simulink model "CommandeClassique"  (R2018a)
settings: Solver=ode4  StartTime=0.0  StopTime=4  FixedStep=1e-5  RelTol=1e-3  EnableMultiTasking=on
values from neighbouring files (symbols this model uses):
  c1 = 0.5176    [Parameters.m]
  c2 = 116    [Parameters.m]
  c3 = 0.4    [Parameters.m]
  c4 = 5    [Parameters.m]
  c5 = 21    [Parameters.m]
  c6 = 0.0068    [Parameters.m]
  Cf = 2e-3    (= 0.002)    [Parameters.m]
  F = (Ft/(G^2))+Fg    (= 0.00731299039781)    [Parameters.m]
  Fsn = 50    [Parameters.m]
  G = 5.4    [Parameters.m]
  J = (Jt/(G^2))+Jg    (= 0.313940329218)    [Parameters.m]
  ki_c = 10*Rr/tou1    (= 620000)    [Parameters.m]
  ki_mppt = J*(wn^2)    (= 10.6826917581)    [Parameters.m]
  ki_p = 1/tou2    (= 100)    [Parameters.m]
  kif = 3*Rf/trf    (= 300)    [Parameters.m]
  kiv_voc = Cf*wn1^2    (= 480.2)    [Parameters.m]
  kp_c = (Lr-((Msr^2)/Ls))/tou1    (= 857.142857143)    [Parameters.m]
  kp_mppt = 2*xi*wn*J    (= 12.8192301097)    [Parameters.m]
  kp_p = tou1/tou2    (= 0.001)    [Parameters.m]
  kpf = 3*Lf/trf    (= 14)    [Parameters.m]
  kpv_voc = 2*ksi1*Cf*wn1    (= 2.548)    [Parameters.m]
  Lf = 0.014    [Parameters.m]
  Lr = 0.081    [Parameters.m]
  Ls = 0.084    [Parameters.m]
  Msr = 0.078    [Parameters.m]
  p = 2    [Parameters.m]
  R = 3    [Parameters.m]
  Rf = 0.3    [Parameters.m]
  rou = 1.225    [Parameters.m]
  s = pi*(R^2)    (= 28.2743338823)    [Parameters.m]
  sigm = (1-((Msr^2)/(Lr*Ls)))    (= 0.10582010582)    [Parameters.m]
  Tr = Lr/Rr    (= 0.13064516129)    [Parameters.m]
  Ts = Ls/Rs    (= 0.184615384615)    [Parameters.m]
  Vs = 380    [Parameters.m]
  Vsn = E/sqrt(3)    [Parameters.m]
  ws = Fsn*pi*2    (= 314.159265359)    [Parameters.m]
undefined symbols (not defined in the file or in its folder): fc
libraries: simulink x26, powerlib_extras x1
settings Model: Creator=HP  LastModifiedBy=Admin
settings DataIOCC: LimitDataPoints=on  SaveFormat=Array  SignalLoggingSaveFormat=ModelDataLogs
settings OptimizationCC: ExpressionDepthLimit=2147483647  LifeSpan=inf
settings DebuggingCC: UnderspecifiedInitializationDetection=Classic  MergeDetectMultiDrivingBlocksExec=none  SolverPrmCheckMsg=warning  FcnCallInpInsideContextMsg=warning  StateNameClashWarn=warning  SFUnexpectedBacktrackingDiag=warning  SFNoUnconditionalDefaultTransitionDiag=warning  SFExecutionAtInitializationDiag=none
settings HardwareCC: ProdBitPerPointer=32  ProdBitPerSizeT=32  ProdBitPerPtrDiffT=32  ProdLargestAtomicFloat=None  ProdIntDivRoundTo=Undefined  ProdEndianess=Unspecified  ProdWordSize=32  ProdHWDeviceType=32-bit Generic
settings ModelReferenceCC: PropagateSignalLabelsOutOfModel=off
settings CodeAppCC: StateflowObjectComments=on
settings GRTTargetCC: TargetLangStandard=C89/C90 (ANSI)  GeneratePreprocessorConditionals=Disable all  CombineOutputUpdateFcns=off  GRTInterface=on
settings ConfigComp: CovMetricSettings=dw  CovHtmlReporting=on  CovSaveCumulativeToWorkspaceVar=on  CovSaveSingleToWorkspaceVar=on  CovExternalEMLEnable=off

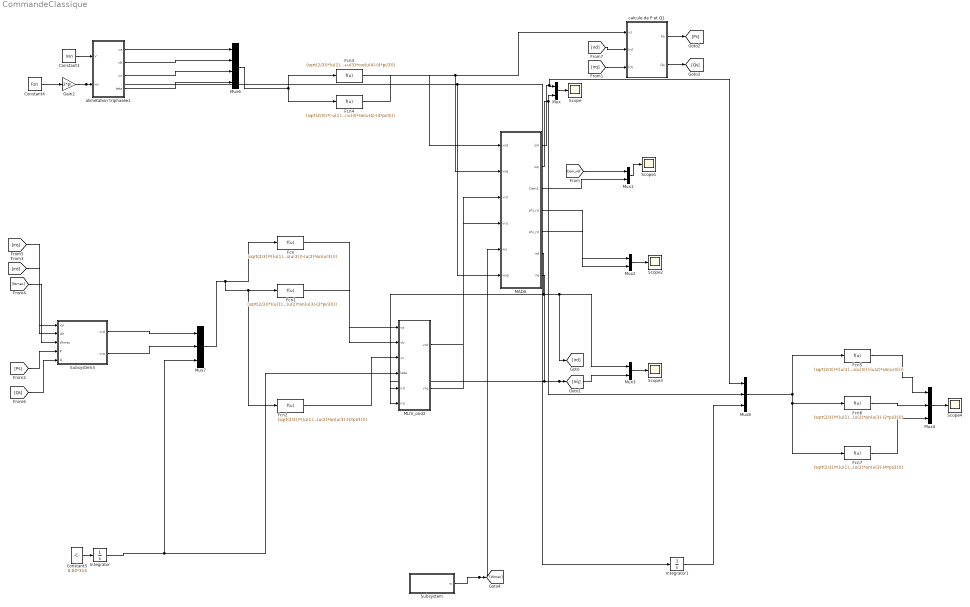
== system CommandeClassique ==
  Constant3 : Constant  Value=Vsn
  Constant4 : Constant  Value=Fsn
  Constant5 : Constant  Value=0.04*314
  Fcn : Fcn  Expr=(sqrt(2/3))*((u(1)*cos(u(3)))-(u(2)*sin(u(3))))
  Fcn1 : Fcn  Expr=(sqrt(2/3))*((u(1)*cos(u(3)-(2*pi/3)))-(u(2)*sin(u(3)-(2*pi/3))))
  Fcn2 : Fcn  Expr=(sqrt(2/3))*((u(1)*cos(u(3)-(4*pi/3)))-(u(2)*sin(u(3)-(4*pi/3))))
  Fcn3 : Fcn  Expr=(sqrt(2/3))*(u(1)*cos(u(4))+u(2)*cos(u(4)-(2*pi/3))+u(3)*cos(u(4)-(4*pi/3)))
  Fcn4 : Fcn  Expr=(sqrt(2/3))*(-u(1)*sin(u(4))-u(2)*sin(u(4)-(2*pi/3))-u(3)*sin(u(4)-(4*pi/3)))
  Fcn5 : Fcn  Expr=(sqrt(2/3))*((u(1)*cos(u(3)))-(u(2)*sin(u(3))))
  Fcn6 : Fcn  Expr=(sqrt(2/3))*((u(1)*cos(u(3)-(2*pi/3)))-(u(2)*sin(u(3)-(2*pi/3))))
  Fcn7 : Fcn  Expr=(sqrt(2/3))*((u(1)*cos(u(3)-(4*pi/3)))-(u(2)*sin(u(3)-(4*pi/3))))
  Gain2 : Gain  Gain=2*pi
  Integrator : Integrator
  Integrator1 : Integrator
  MADA : Subsystem
  MLIV_ond2 : Subsystem
  Mux{,1..3} (4 alike) : Mux  Inputs=2
  Mux4 : Mux  Inputs=3
  Mux6 : Mux
  Mux7 : Mux  Inputs=3
  Mux8 : Mux  Inputs=3
  Scope{,1..4} (5 alike) : Scope
  Subsystem : Subsystem
  Subsystem3 : Subsystem
  alimetation triphasée1 : Subsystem
  calcule de P et Q1 : Subsystem
  wires:
  Constant4/1 -> Gain2/1
  Gain2/1 -> MADA/6(wsp), Integrator1/1, alimetation triphasée1/2(ws)
  Constant3/1 -> alimetation triphasée1/1(V)
  Fcn3/1 -> MADA/1(vsd)
  Fcn4/1 -> calcule de P et Q1/1(vs), MADA/2(vsq)
  [irq] -> Subsystem3/1(iqr)
  [ird] -> Subsystem3/2(idr)
  [Wmec] -> Subsystem3/3(Wmec)
  [Ps] -> Subsystem3/4(P)
  Constant5/1 -> Integrator/1
  MADA/6(ird) -> Mux3/1, [ird], MLIV_ond2/5(ird)
  MADA/7(irq) -> Mux3/2, [irq], MLIV_ond2/6(irq)
  calcule de P et Q1/1(Ps) -> [Ps]
  calcule de P et Q1/2(Qs) -> [Qs]
  Fcn/1 -> MLIV_ond2/1(va)
  Fcn1/1 -> MLIV_ond2/2(vb)
  Fcn2/1 -> MLIV_ond2/3(vc)
  MLIV_ond2/1(vrd) -> MADA/3(vrd)
  MLIV_ond2/2(vrq) -> MADA/4(vrq)
  [ird] -> calcule de P et Q1/2(Ird)
  [irq] -> calcule de P et Q1/3(Irq)
  [Qs] -> Subsystem3/5(Q)
  MADA/3(Cem1) -> Mux1/2
  Subsystem/1(w) -> [Wmec], MADA/5(w1)
  Mux/1 -> Scope/1
  Mux1/1 -> Scope1/1
  [Cem_ref] -> Mux1/1
  Mux2/1 -> Scope2/1
  MADA/5(phi_rd) -> Mux2/1
  MADA/4(phi_rq) -> Mux2/2
  Mux3/1 -> Scope3/1
  Fcn6/1 -> Mux4/2
  Fcn7/1 -> Mux4/3
  Fcn5/1 -> Mux4/1
  Mux4/1 -> Scope4/1
  alimetation triphasée1/3(vc) -> Mux6/3
  alimetation triphasée1/4(teta) -> Mux6/4
  alimetation triphasée1/2(vb) -> Mux6/2
  alimetation triphasée1/1(va) -> Mux6/1
  Mux6/1 -> Fcn3/1, Fcn4/1
  Integrator/1 -> Mux7/3, MLIV_ond2/4(teta)
  Mux7/1 -> Fcn/1, Fcn1/1, Fcn2/1
  Subsystem3/2(vrq) -> Mux7/2
  Subsystem3/1(vrd) -> Mux7/1
  Integrator1/1 -> Mux8/3
  Mux8/1 -> Fcn6/1, Fcn7/1, Fcn5/1
  MADA/2(isq) -> Mux8/2, Mux/2
  MADA/1(isd) -> Mux8/1, Mux/1

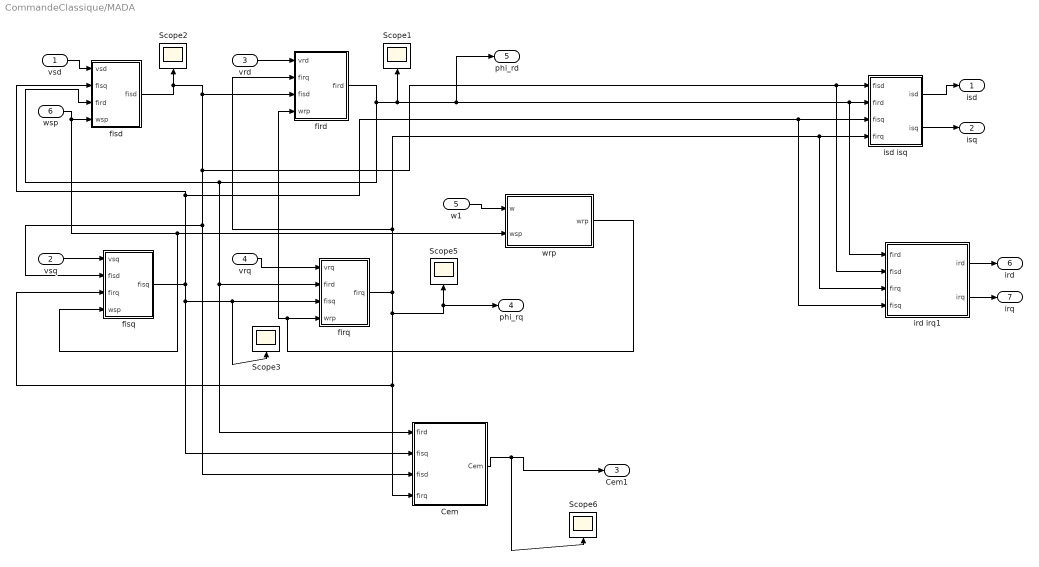
== system CommandeClassique/MADA ==
  vsd : Inport
  vsq : Inport  Port=2
  vrd : Inport  Port=3
  vrq : Inport  Port=4
  w1 : Inport  Port=5
  wsp : Inport  Port=6
  Cem : Subsystem
  Scope{1..3,5..6} (5 alike) : Scope
  fird : Subsystem
  firq : Subsystem
  fisd : Subsystem
  fisq : Subsystem
  ird irq1 : Subsystem
  isd isq : Subsystem
  wrp : Subsystem
  isd : Outport
  isq : Outport  Port=2
  Cem1 : Outport  Port=3
  phi_rq : Outport  Port=4
  phi_rd : Outport  Port=5
  ird : Outport  Port=6
  irq : Outport  Port=7
  wires:
  fisq/1(fisq) -> fisd/2(fisq), isd isq/3(fisq), ird irq1/4(fisq), Cem/2(fisq), firq/3(fisq), Scope3/1
  fird/1(fird) -> fisd/3(fird), firq/2(fird), Cem/1(fird), Scope1/1, phi_rd/1, isd isq/2(fird), ird irq1/1(fird)
  firq/1(firq) -> fird/2(firq), ird irq1/3(firq), isd isq/4(firq), Cem/4(firq), fisq/3(firq), Scope5/1, phi_rq/1
  fisd/1(fisd) -> Scope2/1, Cem/3(fisd), fisq/2(fisd), isd isq/1(fisd), ird irq1/2(fisd), fird/3(fisd)
  Cem/1(Cem) -> Scope6/1, Cem1/1
  vrd/1 -> fird/1(vrd)
  vsd/1 -> fisd/1(vsd)
  isd isq/1(isd) -> isd/1
  wsp/1 -> wrp/2(wsp), fisq/4(wsp), fisd/4(wsp)
  isd isq/2(isq) -> isq/1
  vsq/1 -> fisq/1(vsq)
  vrq/1 -> firq/1(vrq)
  ird irq1/1(ird) -> ird/1
  ird irq1/2(irq) -> irq/1
  wrp/1(wrp) -> firq/4(wrp), fird/4(wrp)
  w1/1 -> wrp/1(w)

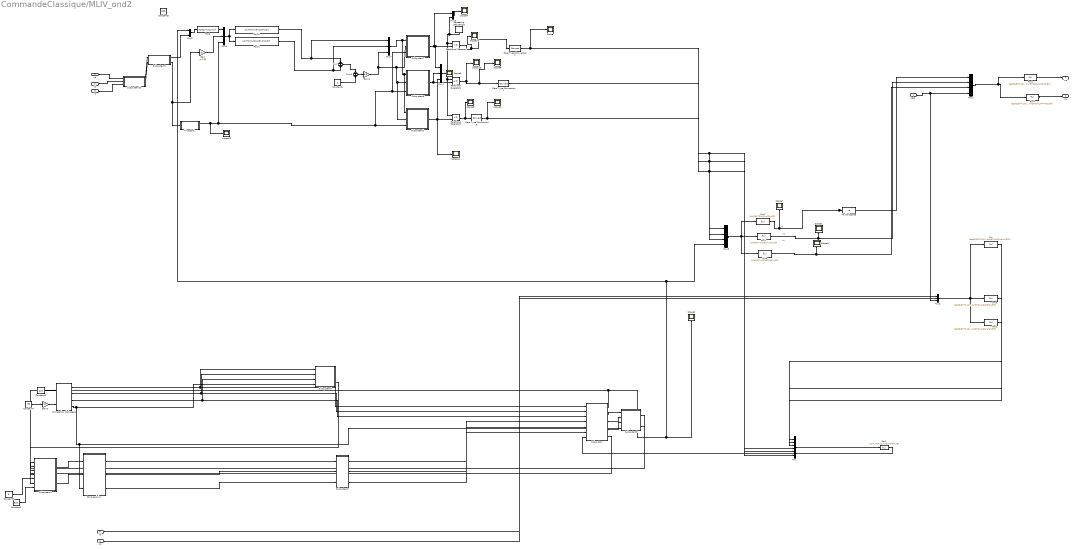
== system CommandeClassique/MLIV_ond2 ==
  note: va
  note: vb
  note: vc
  va : Inport
  vb : Inport  Port=2
  vc : Inport  Port=3
  teta : Inport  Port=4
  ird : Inport  Port=5
  irq : Inport  Port=6
  Constant1 : Constant  Value=525
  Constant2 : Constant  Value=0
  Constant3 : Constant  Value=220
  Constant4 : Constant  Value=50
  Constant5 : Constant  Value=600
  Constant6 : Constant
  Data Type Conversion1 : DataTypeConversion  SaturateOnIntegerOverflow=on  RndMeth=Zero
  Data Type Conversion2 : DataTypeConversion  SaturateOnIntegerOverflow=on  RndMeth=Zero
  Data Type Conversion3 : DataTypeConversion  SaturateOnIntegerOverflow=on  RndMeth=Zero
  Fcn : Fcn  Expr=(sqrt(2/3))*((u(1)*cos(u(3)))-(u(2)*sin(u(3))))
  Fcn1 : Fcn  Expr=u(1)*u(4)+u(2)*u(5)+u(3)*u(6)
  Fcn10 : Fcn  Expr=u(1)*sin((u(3)*pi/3)-u(2))
  Fcn11 : Fcn  Expr=u(1)*(sin(u(2)-(u(3)-1)*pi/3))
  Fcn2 : Fcn  Expr=(sqrt(2/3))*((u(1)*cos(u(3)-(4*pi/3)))-(u(2)*sin(u(3)-(4*pi/3))))
  Fcn3 : Fcn  Expr=(sqrt(2/3))*(u(1)*cos(u(4))+u(2)*cos(u(4)-(2*pi/3))+u(3)*cos(u(4)-(4*pi/3)))
  Fcn4 : Fcn  Expr=(sqrt(2/3))*(-u(1)*sin(u(4))-u(2)*sin(u(4)-(2*pi/3))-u(3)*sin(u(4)-(4*pi/3)))
  Fcn5 : Fcn  Expr=(sqrt(2/3))*((u(1)*cos(u(3)-(2*pi/3)))-(u(2)*sin(u(3)-(2*pi/3))))
  Fcn6 : Fcn  Expr=(u(4)/3)*(2*u(1)-u(2)-u(3))
  Fcn7 : Fcn  Expr=(u(4)/3)*(-u(1)+2*u(2)-u(3))
  Fcn8 : Fcn  Expr=(u(4)/3)*(-u(1)-u(2)+2*u(3))
  Fcn9 : Fcn  Expr=sqrt(2)*(u(2)/u(1))
  Gain : Gain  Gain=pi/180
  Gain1 : Gain  Gain=0.5
  Gain2 : Gain  Gain=2*pi
  Mux : Mux  Inputs=6
  Mux1 : Mux
  Mux{2,4,6..7} (4 alike) : Mux  Inputs=3
  Mux3 : Mux
  Mux5 : Mux  Inputs=2
  Mux8 : Mux  Inputs=2
  N° sector1 : Subsystem
  Relational Operator : RelationalOperator  Operator=<=  OutDataTypeStr=boolean  RndMeth=Nearest
  Relational Operator1 : RelationalOperator  Operator=<=  OutDataTypeStr=boolean  RndMeth=Nearest
  Relational Operator2 : RelationalOperator  Operator=<=  OutDataTypeStr=boolean  RndMeth=Nearest
  Repeating Sequence1 : simulink/Sources/Repeating Sequence  rep_seq_t=[0 1/(4*fc) 1/(2*fc) 3/(4*fc) 1/fc]  rep_seq_y=[0 0.5 1 0.5 0]
  Scope{,1..13} (14 alike) : Scope
  Subsystem : Subsystem
  Subsystem1 : Subsystem
  Subsystem10 : Subsystem
  Subsystem2 : Subsystem
  Subsystem3 : Subsystem
  Subsystem5 : Subsystem
  Subsystem6 : Subsystem
  Subsystem7 : Subsystem
  Subsystem8 : Subsystem
  Subsystem9 : Subsystem
  Sum : Sum  Inputs=+|+
  Sum1 : Sum  Inputs=-|+
  To Workspace : ToWorkspace  VariableName=va  SampleTime=-1
  alimetation triphasée1 : Subsystem
  trans_park_inv : Subsystem
  vrd : Outport
  vrq : Outport  Port=2
  wires:
  Fcn6/1 -> Mux1/1, To Workspace/1, Scope7/1
  Fcn7/1 -> Mux1/2, Scope1/1
  Fcn8/1 -> Mux1/3, Scope3/1
  Mux1/1 -> Fcn3/1, Fcn4/1
  Fcn3/1 -> vrd/1
  Fcn4/1 -> vrq/1
  Fcn1/1 -> Subsystem/7(ich)
  Constant1/1 -> Subsystem1/7(vdc_ref)
  Constant2/1 -> Subsystem1/5(Qref)
  Subsystem3/3(sc) -> Subsystem/6(sc)
  Subsystem3/2(sb) -> Subsystem/5(sb)
  Subsystem3/1(sa) -> Subsystem/4(sa)
  Subsystem1/2(vfq) -> trans_park_inv/2(vrq_ref)
  Subsystem1/1(vfd) -> trans_park_inv/1(vrd_ref)
  trans_park_inv/3(vrc_ref) -> Subsystem3/3(vc)
  trans_park_inv/2(vrb_ref) -> Subsystem3/2(vb)
  trans_park_inv/1(vra_ref) -> Subsystem3/1(va)
  Subsystem/5(Pond) -> Subsystem1/6(Pond)
  Subsystem6/2(vsq) -> Subsystem1/4(vsq)
  Subsystem5/2(ifq) -> Subsystem1/2(ifq)
  Subsystem5/1(ifd) -> Subsystem1/1(ifd)
  alimetation triphasée1/4(teta) -> Subsystem6/4(téta_s), Subsystem5/4(téta_s), trans_park_inv/3(téta_s)
  Subsystem/4(ic) -> Subsystem5/3(ic)
  Subsystem/3(ib) -> Subsystem5/2(ib)
  Subsystem/2(ia) -> Subsystem5/1(ia)
  alimetation triphasée1/3(vc) -> Subsystem/3(ec), Subsystem6/3(vc)
  alimetation triphasée1/2(vb) -> Subsystem/2(eb), Subsystem6/2(vb)
  alimetation triphasée1/1(va) -> Subsystem/1(ea), Subsystem6/1(va)
  Constant3/1 -> alimetation triphasée1/1(V)
  Gain2/1 -> alimetation triphasée1/2(ws)
  Constant4/1 -> Gain2/1
  Mux/1 -> Fcn1/1
  Fcn/1 -> Mux/1
  Fcn5/1 -> Mux/2
  Fcn2/1 -> Mux/3
  ird/1 -> Mux2/1
  irq/1 -> Mux2/2
  Mux2/1 -> Fcn5/1, Fcn2/1, Fcn/1
  teta/1 -> Mux2/3, Mux1/4
  Data Type Conversion2/1 -> Mux3/1, Mux/4, Scope/1
  Data Type Conversion1/1 -> Mux3/2, Mux/5
  Data Type Conversion3/1 -> Mux3/3, Mux/6, Scope9/1
  Mux3/1 -> Fcn7/1, Fcn8/1, Fcn6/1
  Relational Operator/1 -> Data Type Conversion2/1, Scope10/1
  Relational Operator1/1 -> Scope6/1, Data Type Conversion1/1, Scope13/1
  Relational Operator2/1 -> Scope8/1, Data Type Conversion3/1
  Subsystem9/1(module) -> Mux5/2
  Subsystem/1(udc) -> Subsystem1/3(vdc), Mux5/1, Mux3/4, Scope2/1
  Mux5/1 -> Fcn9/1
  Fcn9/1 -> Mux6/1
  Subsystem9/2(téta) -> Gain/1, N° sector1/1(Angle)
  Gain/1 -> Mux6/2
  N° sector1/1(Sector) -> Scope12/1, Subsystem7/3(In3), Subsystem8/3(In3), Subsystem2/3(In3), Mux6/3
  Mux6/1 -> Fcn11/1, Fcn10/1
  Fcn10/1 -> Mux7/1, Sum/1
  Fcn11/1 -> Mux7/2, Sum/2
  Sum/1 -> Sum1/1
  Constant6/1 -> Sum1/2
  Mux7/1 -> Subsystem2/1(Tijo/Ts), Subsystem8/1(Tijo/Ts), Subsystem7/1(Tijo/Ts)
  Sum1/1 -> Gain1/1
  Gain1/1 -> Subsystem2/2(To/Ts), Subsystem8/2(To/Ts), Subsystem7/2(To/Ts), Mux7/3
  Subsystem7/1(TSA/TS) -> Mux4/1, Relational Operator/2, Mux8/1
  Subsystem8/1(TSb/TS) -> Mux4/2, Relational Operator1/2
  Repeating Sequence1/1 -> Mux8/2, Relational Operator/1, Relational Operator1/1, Relational Operator2/1
  Subsystem2/1(TSc/TS) -> Mux4/3, Scope11/1, Relational Operator2/2
  Subsystem10/1(v_alph) -> Subsystem9/1(v_alpha)
  Subsystem10/2(v_beta) -> Subsystem9/2(v_beta)
  vb/1 -> Subsystem10/2(vb)
  va/1 -> Subsystem10/1(va)
  vc/1 -> Subsystem10/3(vc)
  Mux8/1 -> Scope4/1
  Mux4/1 -> Scope5/1

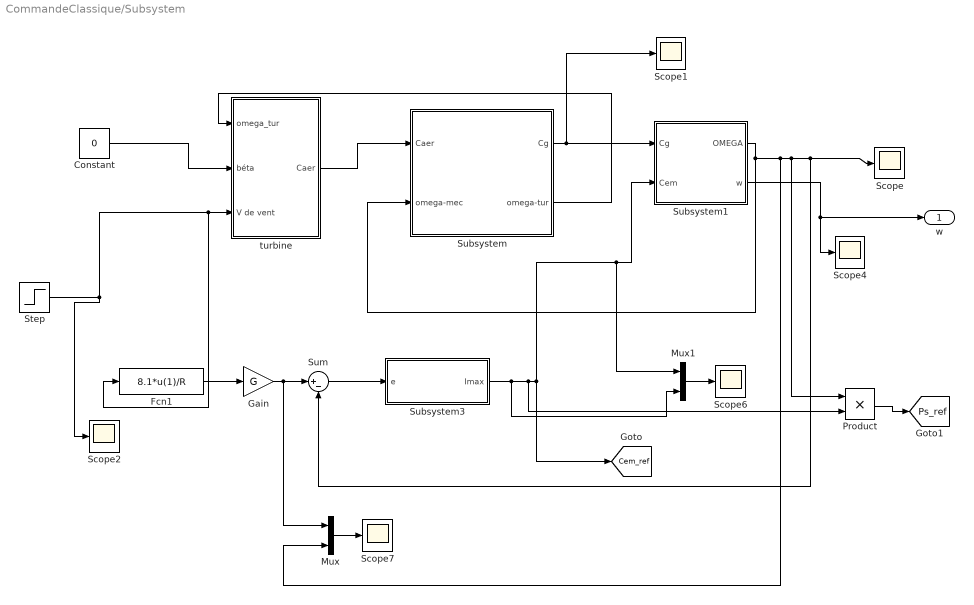
== system CommandeClassique/Subsystem ==
  Constant : Constant  Value=0
  Fcn1 : Fcn  Expr=8.1*u(1)/R
  Gain : Gain  Gain=G
  Mux : Mux  Inputs=2
  Mux1 : Mux  Inputs=2
  Product : Product  RndMeth=Zero
  Scope{,1..2,4,6..7} (6 alike) : Scope
  Step : Step  Time=4  Before=6.5  After=6.5  SampleTime=0
  Subsystem : Subsystem
  Subsystem1 : Subsystem
  Subsystem3 : Subsystem
  Sum : Sum  Inputs=|+-
  turbine : Subsystem
  w : Outport
  tag scope: Cem_ref=global, Ps_ref=global
  wires:
  Constant/1 -> turbine/2(béta)
  turbine/1(Caer) -> Subsystem/1(Caer)
  Subsystem/2(omega-tur) -> turbine/1(omega_tur)
  Step/1 -> Fcn1/1, turbine/3(V de vent), Scope2/1
  Subsystem/1(Cg) -> Scope1/1, Subsystem1/1(Cg)
  Subsystem1/1(OMEGA) -> Subsystem/2(omega-mec), Product/1, Sum/2, Scope/1, Mux/2
  Subsystem1/2(w) -> Scope4/1, w/1
  Fcn1/1 -> Gain/1
  Gain/1 -> Sum/1, Mux/1
  Sum/1 -> Subsystem3/1(e)
  Mux/1 -> Scope7/1
  Subsystem3/1(Imax) -> Product/2, Subsystem1/2(Cem), Mux1/1, [Cem_ref], Mux1/2
  Mux1/1 -> Scope6/1
  Product/1 -> [Ps_ref]

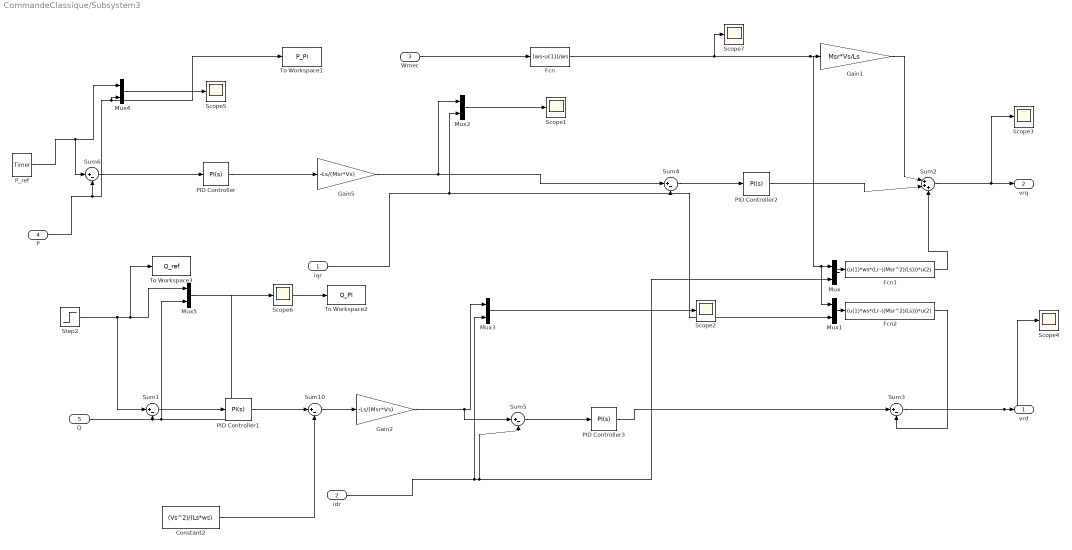
== system CommandeClassique/Subsystem3 ==
  iqr : Inport
  idr : Inport  Port=2
  Wmec : Inport  Port=3
  P : Inport  Port=4
  Q : Inport  Port=5
  Constant2 : Constant  Value=(Vs^2)/(Ls*ws)
  Fcn : Fcn  Expr=(ws-u(1))/ws
  Fcn1 : Fcn  Expr=(u(1)*ws*(Lr-((Msr^2)/Ls)))*u(2)
  Fcn2 : Fcn  Expr=(u(1)*ws*(Lr-((Msr^2)/Ls)))*u(2)
  Gain1 : Gain  Gain=Msr*Vs/Ls
  Gain2 : Gain  Gain=-Ls/(Msr*Vs)
  Gain5 : Gain  Gain=-Ls/(Msr*Vs)
  Mux{,1..5} (6 alike) : Mux  Inputs=2
  PID Controller : simulink/Continuous/PID Controller  Controller=PI  TimeDomain=Continuous-time  SampleTime=-1  IntegratorMethod=Forward Euler  FilterMethod=Forward Euler  Form=Parallel  UseFilter=on  ControllerParametersSource=internal  P=kp_p  I=ki_p  D=0  N=100  InitialConditionSource=internal  InitialConditionForIntegrator=0  InitialConditionForFilter=0  ExternalReset=none  LimitOutput=off  UpperSaturationLimit=inf  LowerSaturationLimit=-inf  LinearizeAsGain=off  AntiWindupMode=none  Kb=1  TrackingMode=off  Kt=1  PParamMin=[]  PParamMax=[]  IParamMin=[]  IParamMax=[]  DParamMin=[]  DParamMax=[]  NParamMin=[]  NParamMax=[]  KbParamMin=[]  KbParamMax=[]  KtParamMin=[]  KtParamMax=[]  POutMin=[]  POutMax=[]  IOutMin=[]  IOutMax=[]  DOutMin=[]  DOutMax=[]  NOutMin=[]  NOutMax=[]  KbOutMin=[]  KbOutMax=[]  KtOutMin=[]  KtOutMax=[]  IntegratorOutMin=[]  IntegratorOutMax=[]  FilterOutMin=[]  FilterOutMax=[]  SumOutMin=[]  SumOutMax=[]  SumI1OutMin=[]  SumI1OutMax=[]  SumI2OutMin=[]  SumI2OutMax=[]  SumI3OutMin=[]  SumI3OutMax=[]  SumDOutMin=[]  SumDOutMax=[]  SaturationOutMin=[]  SaturationOutMax=[]  IntegratorContinuousStateAttributes=''  IntegratorStateMustResolveToSignalObject=off  IntegratorRTWStateStorageClass=Auto  FilterContinuousStateAttributes=''  FilterStateMustResolveToSignalObject=off  FilterRTWStateStorageClass=Auto  DifferentiatorICPrevScaledInput=0  DifferentiatorOutMin=[]  DifferentiatorOutMax=[]  FilterDiffOutCoefMin=[]  FilterDiffOutCoefMax=[]  SumDenOutMin=[]  SumDenOutMax=[]  SumNumOutMin=[]  SumNumOutMax=[]  ReciprocalOutMin=[]  ReciprocalOutMax=[]  DivideOutMin=[]  DivideOutMax=[]  TunerSelectOption=Transfer Function Based (PID Tuner App)
  PID Controller1 : simulink/Continuous/PID Controller  Controller=PI  TimeDomain=Continuous-time  SampleTime=-1  IntegratorMethod=Forward Euler  FilterMethod=Forward Euler  Form=Parallel  UseFilter=on  ControllerParametersSource=internal  P=kp_p  I=ki_p  D=0  N=100  InitialConditionSource=internal  InitialConditionForIntegrator=0  InitialConditionForFilter=0  ExternalReset=none  LimitOutput=off  UpperSaturationLimit=inf  LowerSaturationLimit=-inf  LinearizeAsGain=off  AntiWindupMode=none  Kb=1  TrackingMode=off  Kt=1  PParamMin=[]  PParamMax=[]  IParamMin=[]  IParamMax=[]  DParamMin=[]  DParamMax=[]  NParamMin=[]  NParamMax=[]  KbParamMin=[]  KbParamMax=[]  KtParamMin=[]  KtParamMax=[]  POutMin=[]  POutMax=[]  IOutMin=[]  IOutMax=[]  DOutMin=[]  DOutMax=[]  NOutMin=[]  NOutMax=[]  KbOutMin=[]  KbOutMax=[]  KtOutMin=[]  KtOutMax=[]  IntegratorOutMin=[]  IntegratorOutMax=[]  FilterOutMin=[]  FilterOutMax=[]  SumOutMin=[]  SumOutMax=[]  SumI1OutMin=[]  SumI1OutMax=[]  SumI2OutMin=[]  SumI2OutMax=[]  SumI3OutMin=[]  SumI3OutMax=[]  SumDOutMin=[]  SumDOutMax=[]  SaturationOutMin=[]  SaturationOutMax=[]  IntegratorContinuousStateAttributes=''  IntegratorStateMustResolveToSignalObject=off  IntegratorRTWStateStorageClass=Auto  FilterContinuousStateAttributes=''  FilterStateMustResolveToSignalObject=off  FilterRTWStateStorageClass=Auto  DifferentiatorICPrevScaledInput=0  DifferentiatorOutMin=[]  DifferentiatorOutMax=[]  FilterDiffOutCoefMin=[]  FilterDiffOutCoefMax=[]  SumDenOutMin=[]  SumDenOutMax=[]  SumNumOutMin=[]  SumNumOutMax=[]  ReciprocalOutMin=[]  ReciprocalOutMax=[]  DivideOutMin=[]  DivideOutMax=[]  TunerSelectOption=Transfer Function Based (PID Tuner App)
  PID Controller2 : simulink/Continuous/PID Controller  Controller=PI  TimeDomain=Continuous-time  SampleTime=-1  IntegratorMethod=Forward Euler  FilterMethod=Forward Euler  Form=Parallel  UseFilter=on  ControllerParametersSource=internal  P=kp_c  I=ki_c  D=0  N=100  InitialConditionSource=internal  InitialConditionForIntegrator=0  InitialConditionForFilter=0  ExternalReset=none  LimitOutput=off  UpperSaturationLimit=inf  LowerSaturationLimit=-inf  LinearizeAsGain=off  AntiWindupMode=none  Kb=1  TrackingMode=off  Kt=1  PParamMin=[]  PParamMax=[]  IParamMin=[]  IParamMax=[]  DParamMin=[]  DParamMax=[]  NParamMin=[]  NParamMax=[]  KbParamMin=[]  KbParamMax=[]  KtParamMin=[]  KtParamMax=[]  POutMin=[]  POutMax=[]  IOutMin=[]  IOutMax=[]  DOutMin=[]  DOutMax=[]  NOutMin=[]  NOutMax=[]  KbOutMin=[]  KbOutMax=[]  KtOutMin=[]  KtOutMax=[]  IntegratorOutMin=[]  IntegratorOutMax=[]  FilterOutMin=[]  FilterOutMax=[]  SumOutMin=[]  SumOutMax=[]  SumI1OutMin=[]  SumI1OutMax=[]  SumI2OutMin=[]  SumI2OutMax=[]  SumI3OutMin=[]  SumI3OutMax=[]  SumDOutMin=[]  SumDOutMax=[]  SaturationOutMin=[]  SaturationOutMax=[]  IntegratorContinuousStateAttributes=''  IntegratorStateMustResolveToSignalObject=off  IntegratorRTWStateStorageClass=Auto  FilterContinuousStateAttributes=''  FilterStateMustResolveToSignalObject=off  FilterRTWStateStorageClass=Auto  DifferentiatorICPrevScaledInput=0  DifferentiatorOutMin=[]  DifferentiatorOutMax=[]  FilterDiffOutCoefMin=[]  FilterDiffOutCoefMax=[]  SumDenOutMin=[]  SumDenOutMax=[]  SumNumOutMin=[]  SumNumOutMax=[]  ReciprocalOutMin=[]  ReciprocalOutMax=[]  DivideOutMin=[]  DivideOutMax=[]  TunerSelectOption=Transfer Function Based (PID Tuner App)
  PID Controller3 : simulink/Continuous/PID Controller  Controller=PI  TimeDomain=Continuous-time  SampleTime=-1  IntegratorMethod=Forward Euler  FilterMethod=Forward Euler  Form=Parallel  UseFilter=on  ControllerParametersSource=internal  P=kp_c  I=ki_c  D=0  N=100  InitialConditionSource=internal  InitialConditionForIntegrator=0  InitialConditionForFilter=0  ExternalReset=none  LimitOutput=off  UpperSaturationLimit=inf  LowerSaturationLimit=-inf  LinearizeAsGain=off  AntiWindupMode=none  Kb=1  TrackingMode=off  Kt=1  PParamMin=[]  PParamMax=[]  IParamMin=[]  IParamMax=[]  DParamMin=[]  DParamMax=[]  NParamMin=[]  NParamMax=[]  KbParamMin=[]  KbParamMax=[]  KtParamMin=[]  KtParamMax=[]  POutMin=[]  POutMax=[]  IOutMin=[]  IOutMax=[]  DOutMin=[]  DOutMax=[]  NOutMin=[]  NOutMax=[]  KbOutMin=[]  KbOutMax=[]  KtOutMin=[]  KtOutMax=[]  IntegratorOutMin=[]  IntegratorOutMax=[]  FilterOutMin=[]  FilterOutMax=[]  SumOutMin=[]  SumOutMax=[]  SumI1OutMin=[]  SumI1OutMax=[]  SumI2OutMin=[]  SumI2OutMax=[]  SumI3OutMin=[]  SumI3OutMax=[]  SumDOutMin=[]  SumDOutMax=[]  SaturationOutMin=[]  SaturationOutMax=[]  IntegratorContinuousStateAttributes=''  IntegratorStateMustResolveToSignalObject=off  IntegratorRTWStateStorageClass=Auto  FilterContinuousStateAttributes=''  FilterStateMustResolveToSignalObject=off  FilterRTWStateStorageClass=Auto  DifferentiatorICPrevScaledInput=0  DifferentiatorOutMin=[]  DifferentiatorOutMax=[]  FilterDiffOutCoefMin=[]  FilterDiffOutCoefMax=[]  SumDenOutMin=[]  SumDenOutMax=[]  SumNumOutMin=[]  SumNumOutMax=[]  ReciprocalOutMin=[]  ReciprocalOutMax=[]  DivideOutMin=[]  DivideOutMax=[]  TunerSelectOption=Transfer Function Based (PID Tuner App)
  P_ref : powerlib_extras/Control  Blocks/Timer  t=[0 1 2 3 4]  e=[-5000 -5000 -2000 -3000 -5000]
  Scope{1..7} (7 alike) : Scope
  Step2 : Step  Time=3  After=-2000  SampleTime=0
  Sum{1,3..6,10} (6 alike) : Sum  Inputs=|+-
  Sum2 : Sum  Inputs=|+++
  To Workspace1 : ToWorkspace  VariableName=P_PI  SampleTime=-1
  To Workspace2 : ToWorkspace  VariableName=Q_PI  SampleTime=-1
  To Workspace3 : ToWorkspace  VariableName=Q_ref  SampleTime=-1
  vrd : Outport
  vrq : Outport  Port=2
  wires:
  Fcn/1 -> Scope7/1, Mux1/1, Mux/1, Gain1/1
  Mux5/1 -> Scope6/1
  Mux4/1 -> Scope5/1
  Constant2/1 -> Sum10/2
  PID Controller1/1 -> Sum10/1
  Sum10/1 -> Gain2/1
  Mux3/1 -> Scope2/1
  Mux2/1 -> Scope1/1
  Fcn2/1 -> Sum3/2
  Fcn1/1 -> Sum2/3
  Mux1/1 -> Fcn2/1
  Mux/1 -> Fcn1/1
  Gain1/1 -> Sum2/1
  PID Controller2/1 -> Sum2/2
  PID Controller3/1 -> Sum3/1
  Wmec/1 -> Fcn/1
  Sum3/1 -> Scope4/1, vrd/1
  Sum2/1 -> Scope3/1, vrq/1
  PID Controller/1 -> Gain5/1
  P/1 -> Sum6/2, To Workspace1/1, Mux4/2
  Sum6/1 -> PID Controller/1
  P_ref/1 -> Mux4/1, Sum6/1
  Sum1/1 -> PID Controller1/1
  Q/1 -> Sum1/2, Mux5/2, To Workspace2/1
  Step2/1 -> Sum1/1, To Workspace3/1, Mux5/1
  Sum4/1 -> PID Controller2/1
  iqr/1 -> Mux2/2, Sum4/2, Mux1/2
  Gain5/1 -> Sum4/1, Mux2/1
  Gain2/1 -> Sum5/1, Mux3/1
  idr/1 -> Sum5/2, Mux/2, Mux3/2
  Sum5/1 -> PID Controller3/1

== system CommandeClassique/alimetation triphasée1 ==
  note: teta
  V : Inport
  ws : Inport  Port=2
  Fcn : Fcn  Expr=u[1]*sin(u[2])
  Fcn1 : Fcn  Expr=u[1]*sin(u[2]-(2*pi)/3)
  Fcn2 : Fcn  Expr=u[1]*sin(u[2]-(4*pi)/3)
  Gain : Gain  Gain=sqrt(2)
  Integrator : Integrator
  Mux : Mux  Inputs=2
  va : Outport
  vb : Outport  Port=2
  vc : Outport  Port=3
  teta : Outport  Port=4
  wires:
  Mux/1 -> Fcn/1, Fcn1/1, Fcn2/1
  Gain/1 -> Mux/1
  Integrator/1 -> Mux/2, teta/1
  Fcn/1 -> va/1
  V/1 -> Gain/1
  Fcn1/1 -> vb/1
  Fcn2/1 -> vc/1
  ws/1 -> Integrator/1

== system CommandeClassique/calcule de P et Q1 ==
  vs : Inport
  Ird : Inport  Port=2
  Irq : Inport  Port=3
  Fcn : Fcn  Expr=-((u(1)*Msr/Ls)*u(2))
  Fcn1 : Fcn  Expr=-((u(1)*Msr/Ls)*u(2))+((u(1)^2)/(Ls*ws))
  Mux : Mux  Inputs=2
  Mux1 : Mux  Inputs=2
  Ps : Outport
  Qs : Outport  Port=2
  wires:
  Mux/1 -> Fcn/1
  vs/1 -> Mux/1, Mux1/1
  Mux1/1 -> Fcn1/1
  Irq/1 -> Mux/2
  Ird/1 -> Mux1/2
  Fcn/1 -> Ps/1
  Fcn1/1 -> Qs/1

== system CommandeClassique/MADA/Cem ==
  fird : Inport
  fisq : Inport  Port=2
  fisd : Inport  Port=3
  firq : Inport  Port=4
  Gain1 : Gain  Gain=(1-sigm)/(sigm*Msr)
  Gain2 : Gain  Gain=p
  Product : Product  RndMeth=Zero
  Product1 : Product  RndMeth=Zero
  Sum1 : Sum  Inputs=|+-
  Cem : Outport
  wires:
  Gain1/1 -> Gain2/1
  Sum1/1 -> Gain1/1
  Product1/1 -> Sum1/2
  Product/1 -> Sum1/1
  fird/1 -> Product/1
  fisq/1 -> Product/2
  Gain2/1 -> Cem/1
  fisd/1 -> Product1/1
  firq/1 -> Product1/2

== system CommandeClassique/MADA/fird ==
  vrd : Inport
  firq : Inport  Port=2
  fisd : Inport  Port=3
  wrp : Inport  Port=4
  Gain : Gain  Gain=1/(sigm*Tr)
  Gain12 : Gain  Gain=Msr/(sigm*Tr*Ls)
  Integrator : Integrator  InitialCondition=0.001
  Product1 : Product  RndMeth=Zero
  Sum1 : Sum  Inputs=|+++-
  fird : Outport
  wires:
  Sum1/1 -> Integrator/1
  Gain/1 -> Sum1/4
  Product1/1 -> Sum1/2
  Gain12/1 -> Sum1/3
  vrd/1 -> Sum1/1
  firq/1 -> Product1/1
  wrp/1 -> Product1/2
  fisd/1 -> Gain12/1
  Integrator/1 -> fird/1, Gain/1

== system CommandeClassique/MADA/firq ==
  vrq : Inport
  fird : Inport  Port=2
  fisq : Inport  Port=3
  wrp : Inport  Port=4
  Gain : Gain  Gain=Msr/(sigm*Ls*Tr)
  Gain1 : Gain  Gain=1/(sigm*Tr)
  Integrator : Integrator  InitialCondition=0.001
  Product : Product  RndMeth=Zero
  Sum : Sum  Inputs=|+-+-
  firq : Outport
  wires:
  Product/1 -> Sum/2
  Gain/1 -> Sum/3
  Gain1/1 -> Sum/4
  Sum/1 -> Integrator/1
  Integrator/1 -> firq/1, Gain1/1
  vrq/1 -> Sum/1
  wrp/1 -> Product/2
  fird/1 -> Product/1
  fisq/1 -> Gain/1

== system CommandeClassique/MADA/fisd ==
  vsd : Inport
  fisq : Inport  Port=2
  fird : Inport  Port=3
  wsp : Inport  Port=4
  Gain : Gain  Gain=Msr/(sigm*Lr*Ts)
  Gain1 : Gain  Gain=1/(sigm*Ts)
  Integrator : Integrator
  Product : Product  RndMeth=Zero
  Sum : Sum  Inputs=|+++-
  fisd : Outport
  wires:
  Product/1 -> Sum/2
  Gain/1 -> Sum/3
  Gain1/1 -> Sum/4
  Sum/1 -> Integrator/1
  Integrator/1 -> fisd/1, Gain1/1
  vsd/1 -> Sum/1
  wsp/1 -> Product/2
  fisq/1 -> Product/1
  fird/1 -> Gain/1

== system CommandeClassique/MADA/fisq ==
  vsq : Inport
  fisd : Inport  Port=2
  firq : Inport  Port=3
  wsp : Inport  Port=4
  Gain : Gain  Gain=Msr/(sigm*Lr*Ts)
  Gain1 : Gain  Gain=1/(sigm*Ts)
  Integrator : Integrator
  Product : Product  RndMeth=Zero
  Sum : Sum  Inputs=|+-+-
  fisq : Outport
  wires:
  firq/1 -> Gain/1
  fisd/1 -> Product/1
  wsp/1 -> Product/2
  vsq/1 -> Sum/1
  Integrator/1 -> Gain1/1, fisq/1
  Sum/1 -> Integrator/1
  Gain1/1 -> Sum/4
  Gain/1 -> Sum/3
  Product/1 -> Sum/2

== system CommandeClassique/MADA/ird irq1 ==
  fird : Inport
  fisd : Inport  Port=2
  firq : Inport  Port=3
  fisq : Inport  Port=4
  Gain : Gain  Gain=1/(sigm*Lr)
  Gain1 : Gain  Gain=(1-sigm)/(sigm*Msr)
  Gain2 : Gain  Gain=1/(sigm*Lr)
  Gain3 : Gain  Gain=(1-sigm)/(sigm*Msr)
  Sum : Sum  Inputs=|+-
  Sum1 : Sum  Inputs=|+-
  ird : Outport
  irq : Outport  Port=2
  wires:
  Gain/1 -> Sum/1
  Gain1/1 -> Sum/2
  Gain2/1 -> Sum1/1
  Gain3/1 -> Sum1/2
  fird/1 -> Gain/1
  Sum/1 -> ird/1
  fisd/1 -> Gain1/1
  firq/1 -> Gain2/1
  Sum1/1 -> irq/1
  fisq/1 -> Gain3/1

== system CommandeClassique/MADA/isd isq ==
  fisd : Inport
  fird : Inport  Port=2
  fisq : Inport  Port=3
  firq : Inport  Port=4
  Gain : Gain  Gain=1/(sigm*Ls)
  Gain1 : Gain  Gain=(1-sigm)/(sigm*Msr)
  Gain2 : Gain  Gain=1/(sigm*Ls)
  Gain3 : Gain  Gain=(1-sigm)/(sigm*Msr)
  Sum : Sum  Inputs=|+-
  Sum1 : Sum  Inputs=|+-
  isd : Outport
  isq : Outport  Port=2
  wires:
  Gain/1 -> Sum/1
  Gain1/1 -> Sum/2
  Gain2/1 -> Sum1/1
  Gain3/1 -> Sum1/2
  fisd/1 -> Gain/1
  Sum/1 -> isd/1
  fird/1 -> Gain1/1
  fisq/1 -> Gain2/1
  Sum1/1 -> isq/1
  firq/1 -> Gain3/1

== system CommandeClassique/MADA/wrp ==
  w : Inport
  wsp : Inport  Port=2
  Sum1 : Sum  Inputs=|-+
  wrp : Outport
  wires:
  Sum1/1 -> wrp/1
  w/1 -> Sum1/1
  wsp/1 -> Sum1/2

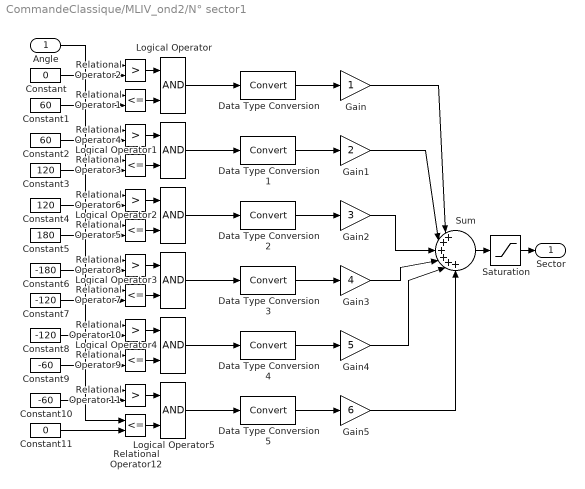
== system CommandeClassique/MLIV_ond2/N° sector1 ==
  Angle : Inport
  Constant : Constant  Value=0
  Constant1 : Constant  Value=60
  Constant10 : Constant  Value=-60
  Constant11 : Constant  Value=0
  Constant2 : Constant  Value=60
  Constant3 : Constant  Value=120
  Constant4 : Constant  Value=120
  Constant5 : Constant  Value=180
  Constant6 : Constant  Value=-180
  Constant7 : Constant  Value=-120
  Constant8 : Constant  Value=-120
  Constant9 : Constant  Value=-60
  Data Type Conversion{,1..5} (6 alike) : DataTypeConversion  SaturateOnIntegerOverflow=on  RndMeth=Zero
  Gain : Gain  SaturateOnIntegerOverflow=on  OutDataTypeStr=Inherit: Same as input  ParamDataTypeStr=Inherit: Same as input
  Gain1 : Gain  Gain=2  SaturateOnIntegerOverflow=on  OutDataTypeStr=Inherit: Same as input  ParamDataTypeStr=Inherit: Same as input
  Gain2 : Gain  Gain=3  SaturateOnIntegerOverflow=on  OutDataTypeStr=Inherit: Same as input  ParamDataTypeStr=Inherit: Same as input
  Gain3 : Gain  Gain=4  SaturateOnIntegerOverflow=on  OutDataTypeStr=Inherit: Same as input  ParamDataTypeStr=Inherit: Same as input
  Gain4 : Gain  Gain=5  SaturateOnIntegerOverflow=on  OutDataTypeStr=Inherit: Same as input  ParamDataTypeStr=Inherit: Same as input
  Gain5 : Gain  Gain=6  SaturateOnIntegerOverflow=on  OutDataTypeStr=Inherit: Same as input  ParamDataTypeStr=Inherit: Same as input
  Logical Operator{,1..5} (6 alike) : Logic
  Relational Operator{1,3,5,7,9,12} (6 alike) : RelationalOperator  Operator=<=  RndMeth=Nearest  InputSameDT=on
  Relational Operator{2,4,6,8,10..11} (6 alike) : RelationalOperator  Operator=>  RndMeth=Nearest  InputSameDT=on
  Saturation : Saturate  UpperLimit=6  LowerLimit=1
  Sum : Sum  Inputs=|++++++  SaturateOnIntegerOverflow=on  InputSameDT=on  OutDataTypeStr=Inherit: Same as first input
  Sector : Outport
  wires:
  Saturation/1 -> Sector/1
  Sum/1 -> Saturation/1
  Gain5/1 -> Sum/6
  Gain4/1 -> Sum/5
  Gain3/1 -> Sum/4
  Gain2/1 -> Sum/3
  Gain1/1 -> Sum/2
  Gain/1 -> Sum/1
  Constant11/1 -> Relational Operator12/2
  Constant10/1 -> Relational Operator11/2
  Logical Operator5/1 -> Data Type Conversion5/1
  Relational Operator12/1 -> Logical Operator5/2
  Relational Operator11/1 -> Logical Operator5/1
  Constant9/1 -> Relational Operator9/2
  Constant8/1 -> Relational Operator10/2
  Logical Operator4/1 -> Data Type Conversion4/1
  Relational Operator9/1 -> Logical Operator4/2
  Relational Operator10/1 -> Logical Operator4/1
  Constant7/1 -> Relational Operator7/2
  Constant6/1 -> Relational Operator8/2
  Logical Operator3/1 -> Data Type Conversion3/1
  Relational Operator7/1 -> Logical Operator3/2
  Relational Operator8/1 -> Logical Operator3/1
  Constant5/1 -> Relational Operator5/2
  Constant4/1 -> Relational Operator6/2
  Logical Operator2/1 -> Data Type Conversion2/1
  Relational Operator5/1 -> Logical Operator2/2
  Relational Operator6/1 -> Logical Operator2/1
  Constant3/1 -> Relational Operator3/2
  Constant2/1 -> Relational Operator4/2
  Logical Operator1/1 -> Data Type Conversion1/1
  Relational Operator3/1 -> Logical Operator1/2
  Relational Operator4/1 -> Logical Operator1/1
  Constant1/1 -> Relational Operator1/2
  Constant/1 -> Relational Operator2/2
  Angle/1 -> Relational Operator12/1, Relational Operator11/1, Relational Operator9/1, Relational Operator10/1, Relational Operator7/1, Relational Operator8/1, Relational Operator5/1, Relational Operator6/1, Relational Operator3/1, Relational Operator4/1, Relational Operator1/1, Relational Operator2/1
  Logical Operator/1 -> Data Type Conversion/1
  Relational Operator1/1 -> Logical Operator/2
  Relational Operator2/1 -> Logical Operator/1
  Data Type Conversion/1 -> Gain/1
  Data Type Conversion1/1 -> Gain1/1
  Data Type Conversion2/1 -> Gain2/1
  Data Type Conversion3/1 -> Gain3/1
  Data Type Conversion4/1 -> Gain4/1
  Data Type Conversion5/1 -> Gain5/1

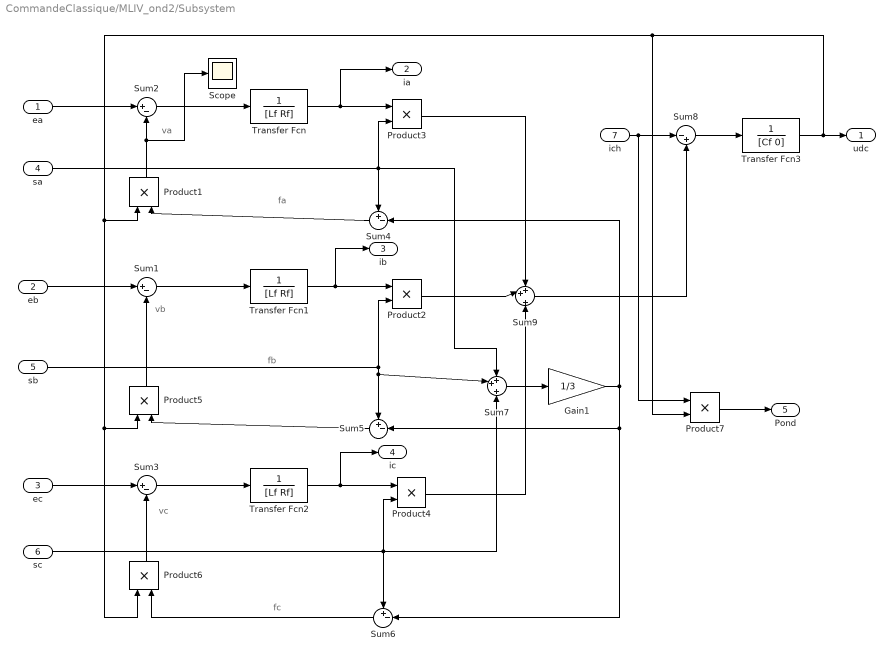
== system CommandeClassique/MLIV_ond2/Subsystem ==
  note: fc
  note: fb
  note: fa
  note: va
  note: vb
  note: vc
  ea : Inport
  eb : Inport  Port=2
  ec : Inport  Port=3
  sa : Inport  Port=4
  sb : Inport  Port=5
  sc : Inport  Port=6
  ich : Inport  Port=7
  Gain1 : Gain  Gain=1/3
  Product{1..7} (7 alike) : Product  RndMeth=Zero
  Scope : Scope
  Sum1 : Sum  Inputs=|+-
  Sum2 : Sum  Inputs=|+-
  Sum3 : Sum  Inputs=|+-
  Sum4 : Sum  Inputs=+-|
  Sum5 : Sum  Inputs=+-|
  Sum6 : Sum  Inputs=+-|
  Sum7 : Sum  Inputs=++|+
  Sum8 : Sum  Inputs=|-+
  Sum9 : Sum  Inputs=++|+
  Transfer Fcn : TransferFcn  Denominator=[Lf Rf]
  Transfer Fcn1 : TransferFcn  Denominator=[Lf Rf]
  Transfer Fcn2 : TransferFcn  Denominator=[Lf Rf]
  Transfer Fcn3 : TransferFcn  Denominator=[Cf 0]
  udc : Outport
  ia : Outport  Port=2
  ib : Outport  Port=3
  ic : Outport  Port=4
  Pond : Outport  Port=5
  wires:
  ea/1 -> Sum2/1
  eb/1 -> Sum1/1
  ec/1 -> Sum3/1
  Sum2/1 -> Transfer Fcn/1
  Sum1/1 -> Transfer Fcn1/1
  Sum3/1 -> Transfer Fcn2/1
  Transfer Fcn/1 -> Product3/1, ia/1
  Transfer Fcn1/1 -> Product2/1, ib/1
  Transfer Fcn2/1 -> Product4/1, ic/1
  Sum7/1 -> Gain1/1
  Gain1/1 -> Sum4/2, Sum5/2, Sum6/2
  sb/1 -> Product2/2, Sum7/2, Sum5/1
  sa/1 -> Product3/2, Sum7/1, Sum4/1
  sc/1 -> Product4/2, Sum7/3, Sum6/1
  Sum6/1 -> Product6/2
  Sum4/1 -> Product1/2
  Sum5/1 -> Product5/2
  Product1/1 -> Sum2/2, Scope/1
  Product5/1 -> Sum1/2
  Product6/1 -> Sum3/2
  Sum8/1 -> Transfer Fcn3/1
  Product3/1 -> Sum9/1
  Product2/1 -> Sum9/2
  Product4/1 -> Sum9/3
  Sum9/1 -> Sum8/2
  Transfer Fcn3/1 -> udc/1, Product1/1, Product5/1, Product6/1, Product7/2
  ich/1 -> Sum8/1, Product7/1
  Product7/1 -> Pond/1

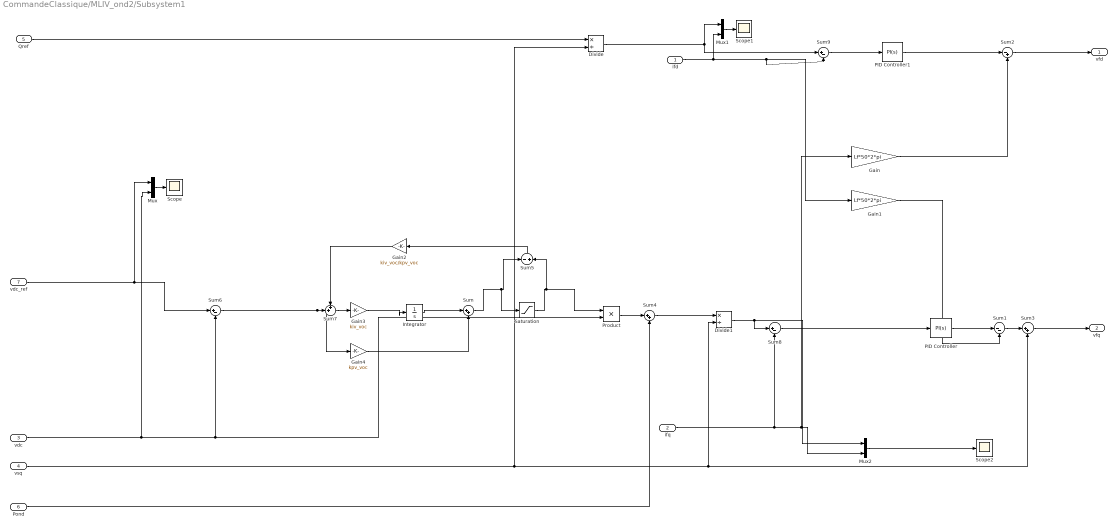
== system CommandeClassique/MLIV_ond2/Subsystem1 ==
  ifd : Inport
  ifq : Inport  Port=2
  vdc : Inport  Port=3
  vsq : Inport  Port=4
  Qref : Inport  Port=5
  Pond : Inport  Port=6
  vdc_ref : Inport  Port=7
  Divide : Product  Inputs=*/
  Divide1 : Product  Inputs=*/
  Gain : Gain  Gain=Lf*50*2*pi
  Gain1 : Gain  Gain=Lf*50*2*pi
  Gain2 : Gain  Gain=kiv_voc/kpv_voc
  Gain3 : Gain  Gain=kiv_voc
  Gain4 : Gain  Gain=kpv_voc
  Integrator : Integrator
  Mux : Mux  Inputs=2
  Mux1 : Mux  Inputs=2
  Mux2 : Mux  Inputs=2
  PID Controller : simulink/Continuous/PID Controller  Controller=PI  TimeDomain=Continuous-time  SampleTime=-1  IntegratorMethod=Forward Euler  FilterMethod=Forward Euler  Form=Parallel  UseFilter=on  ControllerParametersSource=internal  P=kpf  I=kif  D=0  N=100  InitialConditionSource=internal  InitialConditionForIntegrator=0  InitialConditionForFilter=0  ExternalReset=none  LimitOutput=off  UpperSaturationLimit=inf  LowerSaturationLimit=-inf  LinearizeAsGain=off  AntiWindupMode=none  Kb=1  TrackingMode=off  Kt=1  PParamMin=[]  PParamMax=[]  IParamMin=[]  IParamMax=[]  DParamMin=[]  DParamMax=[]  NParamMin=[]  NParamMax=[]  KbParamMin=[]  KbParamMax=[]  KtParamMin=[]  KtParamMax=[]  POutMin=[]  POutMax=[]  IOutMin=[]  IOutMax=[]  DOutMin=[]  DOutMax=[]  NOutMin=[]  NOutMax=[]  KbOutMin=[]  KbOutMax=[]  KtOutMin=[]  KtOutMax=[]  IntegratorOutMin=[]  IntegratorOutMax=[]  FilterOutMin=[]  FilterOutMax=[]  SumOutMin=[]  SumOutMax=[]  SumI1OutMin=[]  SumI1OutMax=[]  SumI2OutMin=[]  SumI2OutMax=[]  SumI3OutMin=[]  SumI3OutMax=[]  SumDOutMin=[]  SumDOutMax=[]  SaturationOutMin=[]  SaturationOutMax=[]  IntegratorContinuousStateAttributes=''  IntegratorStateMustResolveToSignalObject=off  IntegratorRTWStateStorageClass=Auto  FilterContinuousStateAttributes=''  FilterStateMustResolveToSignalObject=off  FilterRTWStateStorageClass=Auto  DifferentiatorICPrevScaledInput=0  DifferentiatorOutMin=[]  DifferentiatorOutMax=[]  FilterDiffOutCoefMin=[]  FilterDiffOutCoefMax=[]  SumDenOutMin=[]  SumDenOutMax=[]  SumNumOutMin=[]  SumNumOutMax=[]  ReciprocalOutMin=[]  ReciprocalOutMax=[]  DivideOutMin=[]  DivideOutMax=[]  TunerSelectOption=Transfer Function Based (PID Tuner App)
  PID Controller1 : simulink/Continuous/PID Controller  Controller=PI  TimeDomain=Continuous-time  SampleTime=-1  IntegratorMethod=Forward Euler  FilterMethod=Forward Euler  Form=Parallel  UseFilter=on  ControllerParametersSource=internal  P=kpf  I=kif  D=0  N=100  InitialConditionSource=internal  InitialConditionForIntegrator=0  InitialConditionForFilter=0  ExternalReset=none  LimitOutput=off  UpperSaturationLimit=inf  LowerSaturationLimit=-inf  LinearizeAsGain=off  AntiWindupMode=none  Kb=1  TrackingMode=off  Kt=1  PParamMin=[]  PParamMax=[]  IParamMin=[]  IParamMax=[]  DParamMin=[]  DParamMax=[]  NParamMin=[]  NParamMax=[]  KbParamMin=[]  KbParamMax=[]  KtParamMin=[]  KtParamMax=[]  POutMin=[]  POutMax=[]  IOutMin=[]  IOutMax=[]  DOutMin=[]  DOutMax=[]  NOutMin=[]  NOutMax=[]  KbOutMin=[]  KbOutMax=[]  KtOutMin=[]  KtOutMax=[]  IntegratorOutMin=[]  IntegratorOutMax=[]  FilterOutMin=[]  FilterOutMax=[]  SumOutMin=[]  SumOutMax=[]  SumI1OutMin=[]  SumI1OutMax=[]  SumI2OutMin=[]  SumI2OutMax=[]  SumI3OutMin=[]  SumI3OutMax=[]  SumDOutMin=[]  SumDOutMax=[]  SaturationOutMin=[]  SaturationOutMax=[]  IntegratorContinuousStateAttributes=''  IntegratorStateMustResolveToSignalObject=off  IntegratorRTWStateStorageClass=Auto  FilterContinuousStateAttributes=''  FilterStateMustResolveToSignalObject=off  FilterRTWStateStorageClass=Auto  DifferentiatorICPrevScaledInput=0  DifferentiatorOutMin=[]  DifferentiatorOutMax=[]  FilterDiffOutCoefMin=[]  FilterDiffOutCoefMax=[]  SumDenOutMin=[]  SumDenOutMax=[]  SumNumOutMin=[]  SumNumOutMax=[]  ReciprocalOutMin=[]  ReciprocalOutMax=[]  DivideOutMin=[]  DivideOutMax=[]  TunerSelectOption=Transfer Function Based (PID Tuner App)
  Product : Product  RndMeth=Zero
  Saturation : Saturate  UpperLimit=50  LowerLimit=-50
  Scope : Scope
  Scope1 : Scope
  Scope2 : Scope
  Sum : Sum  Inputs=|++
  Sum1 : Sum  Inputs=|--
  Sum2 : Sum  Inputs=|-+
  Sum3 : Sum  Inputs=|++
  Sum4 : Sum  Inputs=|++
  Sum5 : Sum  Inputs=-|+
  Sum6 : Sum  Inputs=|+-
  Sum7 : Sum  Inputs=++|
  Sum8 : Sum  Inputs=|+-
  Sum9 : Sum  Inputs=|+-
  vfd : Outport
  vfq : Outport  Port=2
  wires:
  Sum3/1 -> vfq/1
  Sum2/1 -> vfd/1
  vsq/1 -> Divide/2, Sum3/2, Divide1/2
  Sum1/1 -> Sum3/1
  PID Controller1/1 -> Sum2/1
  PID Controller/1 -> Sum1/1
  Gain/1 -> Sum2/2
  Gain1/1 -> Sum1/2
  Qref/1 -> Divide/1
  Sum4/1 -> Divide1/1
  Pond/1 -> Sum4/2
  Product/1 -> Sum4/1
  Mux/1 -> Scope/1
  Mux1/1 -> Scope1/1
  Mux2/1 -> Scope2/1
  Saturation/1 -> Product/1, Sum5/2
  Sum5/1 -> Gain2/1
  Sum7/1 -> Gain3/1
  Gain4/1 -> Sum/2
  Integrator/1 -> Sum/1
  Gain3/1 -> Integrator/1
  Sum6/1 -> Sum7/2, Gain4/1
  Gain2/1 -> Sum7/1
  Sum/1 -> Saturation/1, Sum5/1
  vdc/1 -> Sum6/2, Product/2, Mux/2
  vdc_ref/1 -> Sum6/1, Mux/1
  Sum8/1 -> PID Controller/1
  ifq/1 -> Sum8/2, Gain/1, Mux2/2
  Divide1/1 -> Sum8/1, Mux2/1
  Divide/1 -> Sum9/1, Mux1/1
  ifd/1 -> Sum9/2, Gain1/1, Mux1/2
  Sum9/1 -> PID Controller1/1

== system CommandeClassique/MLIV_ond2/Subsystem10 ==
  va : Inport
  vb : Inport  Port=2
  vc : Inport  Port=3
  Fcn : Fcn  Expr=sqrt(2/3)*(u(1)-(1/2)*u(2)-(1/2)*u(3))
  Fcn1 : Fcn  Expr=sqrt(2/3)*(((sqrt(3)/2)*u(2))-((sqrt(3)/2)*u(3)))
  Mux : Mux  Inputs=3
  v_alph : Outport
  v_beta : Outport  Port=2
  wires:
  Fcn1/1 -> v_beta/1
  Fcn/1 -> v_alph/1
  Mux/1 -> Fcn1/1, Fcn/1
  vc/1 -> Mux/3
  vb/1 -> Mux/2
  va/1 -> Mux/1

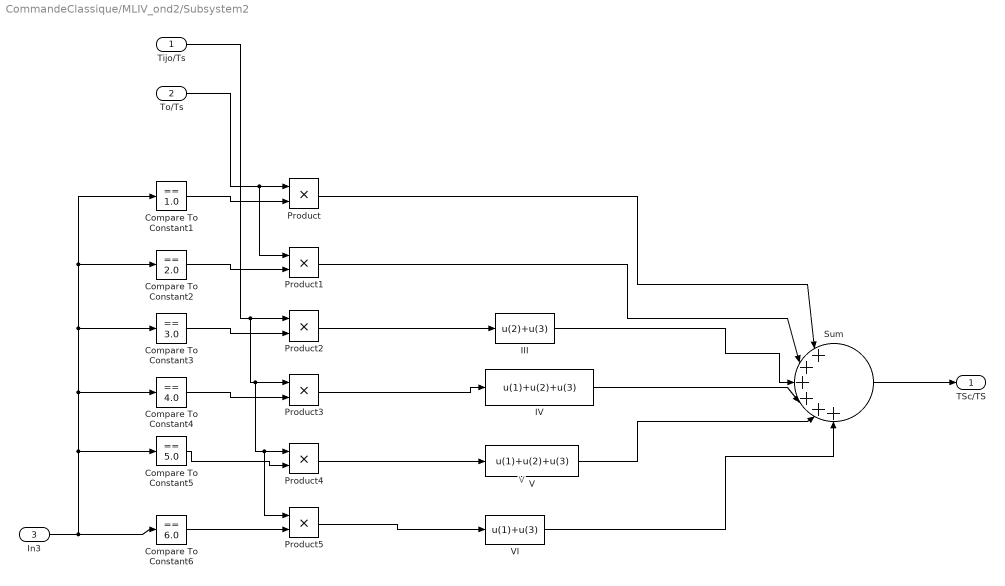
== system CommandeClassique/MLIV_ond2/Subsystem2 ==
  note: V
  Tijo/Ts : Inport
  To/Ts : Inport  Port=2
  In3 : Inport  Port=3
  Compare To Constant1 : simulink/Logic and Bit Operations/Compare To Constant  relop===  const=1.0  OutDataTypeStr=uint8
  Compare To Constant2 : simulink/Logic and Bit Operations/Compare To Constant  relop===  const=2.0  OutDataTypeStr=uint8
  Compare To Constant3 : simulink/Logic and Bit Operations/Compare To Constant  relop===  const=3.0  OutDataTypeStr=uint8
  Compare To Constant4 : simulink/Logic and Bit Operations/Compare To Constant  relop===  const=4.0  OutDataTypeStr=uint8
  Compare To Constant5 : simulink/Logic and Bit Operations/Compare To Constant  relop===  const=5.0  OutDataTypeStr=uint8
  Compare To Constant6 : simulink/Logic and Bit Operations/Compare To Constant  relop===  const=6.0  OutDataTypeStr=uint8
  III : Fcn  Expr=u(2)+u(3)
  IV : Fcn  Expr=u(1)+u(2)+u(3)
  Product{,1..5} (6 alike) : Product  RndMeth=Zero
  Sum : Sum  Inputs=|++++++
  V : Fcn  Expr=u(1)+u(2)+u(3)
  VI : Fcn  Expr=u(1)+u(3)
  TSc/TS : Outport
  wires:
  Sum/1 -> TSc/TS/1
  VI/1 -> Sum/6
  V/1 -> Sum/5
  Tijo/Ts/1 -> Product5/1, Product4/1, Product3/1, Product2/1
  To/Ts/1 -> Product1/1, Product/1
  Product5/1 -> VI/1
  Product4/1 -> V/1
  Compare To Constant6/1 -> Product5/2
  Compare To Constant5/1 -> Product4/2
  Compare To Constant4/1 -> Product3/2
  Product3/1 -> IV/1
  Compare To Constant3/1 -> Product2/2
  Product2/1 -> III/1
  Compare To Constant2/1 -> Product1/2
  Product1/1 -> Sum/2
  Compare To Constant1/1 -> Product/2
  Product/1 -> Sum/1
  In3/1 -> Compare To Constant6/1, Compare To Constant5/1, Compare To Constant4/1, Compare To Constant3/1, Compare To Constant2/1, Compare To Constant1/1
  III/1 -> Sum/3
  IV/1 -> Sum/4

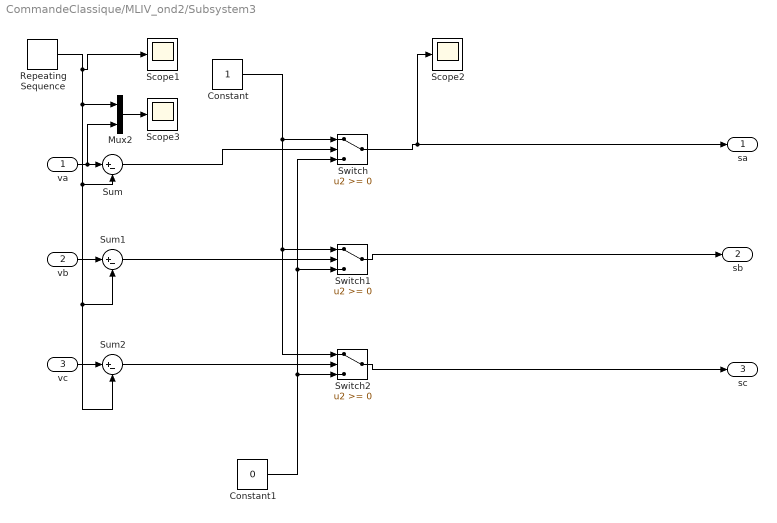
== system CommandeClassique/MLIV_ond2/Subsystem3 ==
  va : Inport
  vb : Inport  Port=2
  vc : Inport  Port=3
  Constant : Constant
  Constant1 : Constant  Value=0
  Mux2 : Mux  Inputs=2
  Repeating Sequence : simulink/Sources/Repeating Sequence  rep_seq_t=[0 1/(4*2050) 1/(2*2050) 3/(4*2050) 1/2050]  rep_seq_y=[0 1200 0 -1200 0]
  Scope1 : Scope
  Scope2 : Scope
  Scope3 : Scope
  Sum : Sum  Inputs=|+-
  Sum1 : Sum  Inputs=|+-
  Sum2 : Sum  Inputs=|+-
  Switch : Switch
  Switch1 : Switch
  Switch2 : Switch
  sa : Outport
  sb : Outport  Port=2
  sc : Outport  Port=3
  wires:
  Sum/1 -> Switch/2
  Sum1/1 -> Switch1/2
  Sum2/1 -> Switch2/2
  Constant/1 -> Switch/1, Switch1/1, Switch2/1
  Constant1/1 -> Switch2/3, Switch1/3, Switch/3
  Repeating Sequence/1 -> Scope1/1, Sum/2, Sum1/2, Sum2/2, Mux2/1
  Switch/1 -> Scope2/1, sa/1
  va/1 -> Sum/1, Mux2/2
  Switch1/1 -> sb/1
  vb/1 -> Sum1/1
  vc/1 -> Sum2/1
  Switch2/1 -> sc/1
  Mux2/1 -> Scope3/1

== system CommandeClassique/MLIV_ond2/Subsystem5 ==
  ia : Inport
  ib : Inport  Port=2
  ic : Inport  Port=3
  téta_s : Inport  Port=4
  Fcn1 : Fcn  Expr=(sqrt(2/3))*(u(1)*cos(u(4))+u(2)*cos(u(4)-(2*pi/3))+u(3)*cos(u(4)-(4*pi/3)))
  Fcn2 : Fcn  Expr=(sqrt(2/3))*(-u(1)*sin(u(4))-u(2)*sin(u(4)-(2*pi/3))-u(3)*sin(u(4)-(4*pi/3)))
  Mux2 : Mux
  Scope2 : Scope
  ifd : Outport
  ifq : Outport  Port=2
  wires:
  ia/1 -> Mux2/1
  ib/1 -> Mux2/2
  ic/1 -> Mux2/3
  Mux2/1 -> Fcn2/1, Fcn1/1
  Fcn1/1 -> ifd/1, Scope2/1
  téta_s/1 -> Mux2/4
  Fcn2/1 -> ifq/1

== system CommandeClassique/MLIV_ond2/Subsystem6 ==
  va : Inport
  vb : Inport  Port=2
  vc : Inport  Port=3
  téta_s : Inport  Port=4
  Fcn1 : Fcn  Expr=(sqrt(2/3))*(u(1)*cos(u(4))+u(2)*cos(u(4)-(2*pi/3))+u(3)*cos(u(4)-(4*pi/3)))
  Fcn2 : Fcn  Expr=(sqrt(2/3))*(-u(1)*sin(u(4))-u(2)*sin(u(4)-(2*pi/3))-u(3)*sin(u(4)-(4*pi/3)))
  Mux2 : Mux
  Scope2 : Scope
  vsd : Outport
  vsq : Outport  Port=2
  wires:
  Fcn2/1 -> vsq/1
  téta_s/1 -> Mux2/4
  Fcn1/1 -> Scope2/1, vsd/1
  Mux2/1 -> Fcn1/1, Fcn2/1
  vc/1 -> Mux2/3
  vb/1 -> Mux2/2
  va/1 -> Mux2/1

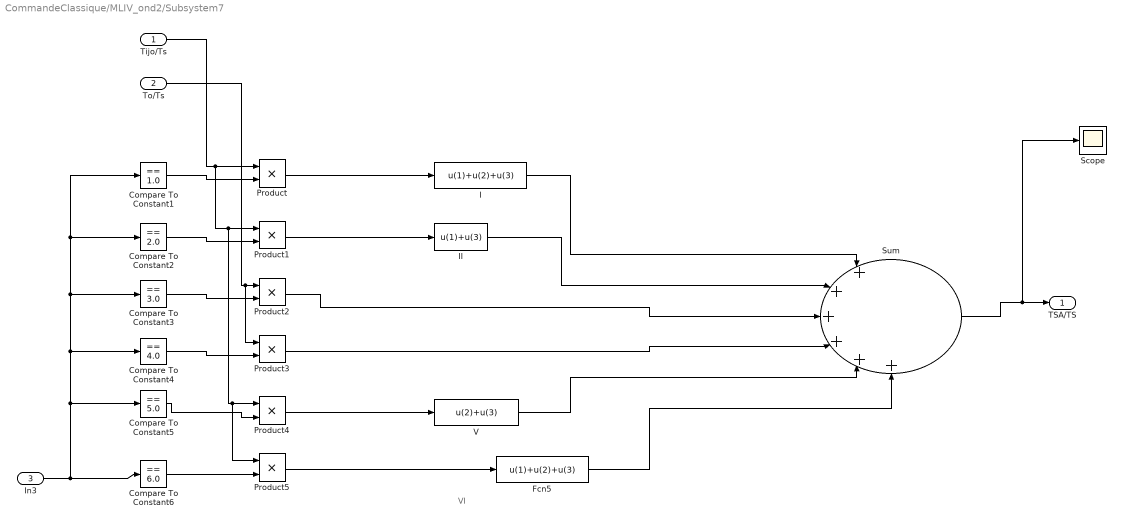
== system CommandeClassique/MLIV_ond2/Subsystem7 ==
  note: VI
  Tijo/Ts : Inport
  To/Ts : Inport  Port=2
  In3 : Inport  Port=3
  Compare To Constant1 : simulink/Logic and Bit Operations/Compare To Constant  relop===  const=1.0  OutDataTypeStr=uint8
  Compare To Constant2 : simulink/Logic and Bit Operations/Compare To Constant  relop===  const=2.0  OutDataTypeStr=uint8
  Compare To Constant3 : simulink/Logic and Bit Operations/Compare To Constant  relop===  const=3.0  OutDataTypeStr=uint8
  Compare To Constant4 : simulink/Logic and Bit Operations/Compare To Constant  relop===  const=4.0  OutDataTypeStr=uint8
  Compare To Constant5 : simulink/Logic and Bit Operations/Compare To Constant  relop===  const=5.0  OutDataTypeStr=uint8
  Compare To Constant6 : simulink/Logic and Bit Operations/Compare To Constant  relop===  const=6.0  OutDataTypeStr=uint8
  Fcn5 : Fcn  Expr=u(1)+u(2)+u(3)
  I : Fcn  Expr=u(1)+u(2)+u(3)
  II : Fcn  Expr=u(1)+u(3)
  Product{,1..5} (6 alike) : Product  RndMeth=Zero
  Scope : Scope
  Sum : Sum  Inputs=|++++++
  V : Fcn  Expr=u(2)+u(3)
  TSA/TS : Outport
  wires:
  Sum/1 -> Scope/1, TSA/TS/1
  Fcn5/1 -> Sum/6
  V/1 -> Sum/5
  II/1 -> Sum/2
  I/1 -> Sum/1
  Product5/1 -> Fcn5/1
  Product4/1 -> V/1
  Compare To Constant6/1 -> Product5/2
  Compare To Constant5/1 -> Product4/2
  To/Ts/1 -> Product3/1, Product2/1
  Compare To Constant4/1 -> Product3/2
  Product3/1 -> Sum/4
  Compare To Constant3/1 -> Product2/2
  Product2/1 -> Sum/3
  Compare To Constant2/1 -> Product1/2
  Product1/1 -> II/1
  Compare To Constant1/1 -> Product/2
  Tijo/Ts/1 -> Product5/1, Product4/1, Product1/1, Product/1
  Product/1 -> I/1
  In3/1 -> Compare To Constant6/1, Compare To Constant5/1, Compare To Constant4/1, Compare To Constant3/1, Compare To Constant2/1, Compare To Constant1/1

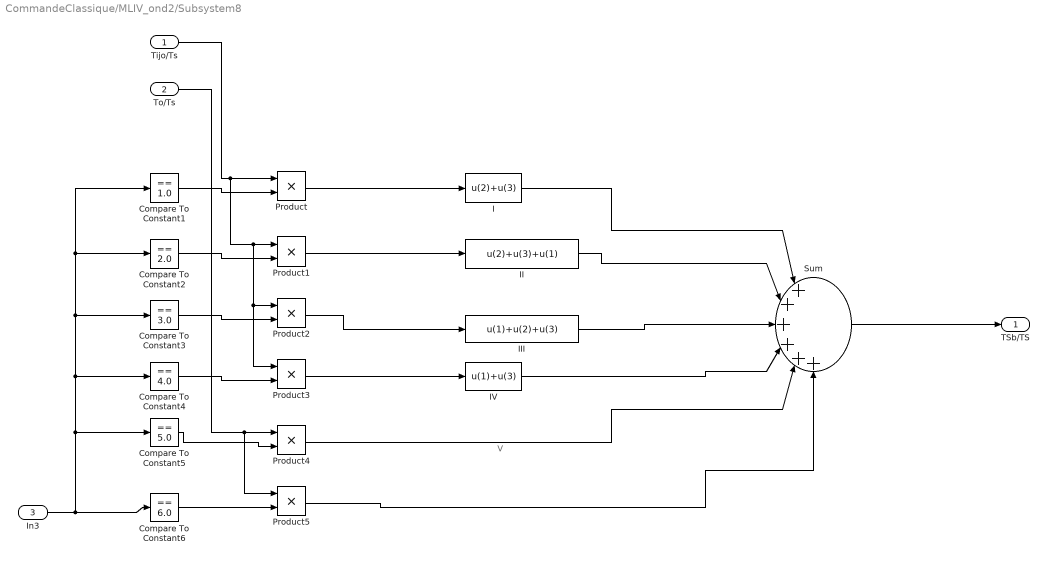
== system CommandeClassique/MLIV_ond2/Subsystem8 ==
  note: V
  Tijo/Ts : Inport
  To/Ts : Inport  Port=2
  In3 : Inport  Port=3
  Compare To Constant1 : simulink/Logic and Bit Operations/Compare To Constant  relop===  const=1.0  OutDataTypeStr=uint8
  Compare To Constant2 : simulink/Logic and Bit Operations/Compare To Constant  relop===  const=2.0  OutDataTypeStr=uint8
  Compare To Constant3 : simulink/Logic and Bit Operations/Compare To Constant  relop===  const=3.0  OutDataTypeStr=uint8
  Compare To Constant4 : simulink/Logic and Bit Operations/Compare To Constant  relop===  const=4.0  OutDataTypeStr=uint8
  Compare To Constant5 : simulink/Logic and Bit Operations/Compare To Constant  relop===  const=5.0  OutDataTypeStr=uint8
  Compare To Constant6 : simulink/Logic and Bit Operations/Compare To Constant  relop===  const=6.0  OutDataTypeStr=uint8
  I : Fcn  Expr=u(2)+u(3)
  II : Fcn  Expr=u(2)+u(3)+u(1)
  III : Fcn  Expr=u(1)+u(2)+u(3)
  IV : Fcn  Expr=u(1)+u(3)
  Product{,1..5} (6 alike) : Product  RndMeth=Zero
  Sum : Sum  Inputs=|++++++
  TSb/TS : Outport
  wires:
  III/1 -> Sum/3
  Sum/1 -> TSb/TS/1
  To/Ts/1 -> Product5/1, Product4/1
  IV/1 -> Sum/4
  In3/1 -> Compare To Constant1/1, Compare To Constant2/1, Compare To Constant3/1, Compare To Constant4/1, Compare To Constant5/1, Compare To Constant6/1
  Product/1 -> I/1
  Tijo/Ts/1 -> Product3/1, Product2/1, Product1/1, Product/1
  Compare To Constant1/1 -> Product/2
  Product1/1 -> II/1
  Compare To Constant2/1 -> Product1/2
  Product2/1 -> III/1
  Compare To Constant3/1 -> Product2/2
  Product3/1 -> IV/1
  Compare To Constant4/1 -> Product3/2
  Compare To Constant5/1 -> Product4/2
  Compare To Constant6/1 -> Product5/2
  Product4/1 -> Sum/5
  Product5/1 -> Sum/6
  I/1 -> Sum/1
  II/1 -> Sum/2

== system CommandeClassique/MLIV_ond2/Subsystem9 ==
  v_alpha : Inport
  v_beta : Inport  Port=2
  Fcn : Fcn  Expr=sqrt((u(1)^2)+(u(2)^2))
  Fcn1 : Fcn  Expr=atan2(u(2),u(1))
  Gain : Gain  Gain=180/pi
  Mux : Mux  Inputs=2
  Mux1 : Mux  Inputs=2
  module : Outport
  téta : Outport  Port=2
  wires:
  Gain/1 -> téta/1
  Fcn1/1 -> Gain/1
  Mux1/1 -> Fcn1/1
  Fcn/1 -> module/1
  v_beta/1 -> Mux1/2, Mux/2
  v_alpha/1 -> Mux1/1, Mux/1
  Mux/1 -> Fcn/1

== system CommandeClassique/MLIV_ond2/alimetation triphasée1 ==
  note: teta
  V : Inport
  ws : Inport  Port=2
  Fcn : Fcn  Expr=u[1]*sin(u[2])
  Fcn1 : Fcn  Expr=u[1]*sin(u[2]-(2*pi)/3)
  Fcn2 : Fcn  Expr=u[1]*sin(u[2]-(4*pi)/3)
  Gain : Gain  Gain=sqrt(2)
  Integrator : Integrator
  Mux : Mux  Inputs=2
  va : Outport
  vb : Outport  Port=2
  vc : Outport  Port=3
  teta : Outport  Port=4
  wires:
  Mux/1 -> Fcn/1, Fcn1/1, Fcn2/1
  Gain/1 -> Mux/1
  Integrator/1 -> Mux/2, teta/1
  Fcn/1 -> va/1
  V/1 -> Gain/1
  Fcn1/1 -> vb/1
  Fcn2/1 -> vc/1
  ws/1 -> Integrator/1

== system CommandeClassique/MLIV_ond2/trans_park_inv ==
  vrd_ref : Inport
  vrq_ref : Inport  Port=2
  téta_s : Inport  Port=3
  Fcn : Fcn  Expr=(sqrt(2/3))*((u(1)*cos(u(3)))-(u(2)*sin(u(3))))
  Fcn1 : Fcn  Expr=(sqrt(2/3))*((u(1)*cos(u(3)-(2*pi/3)))-(u(2)*sin(u(3)-(2*pi/3))))
  Fcn2 : Fcn  Expr=(sqrt(2/3))*((u(1)*cos(u(3)-(4*pi/3)))-(u(2)*sin(u(3)-(4*pi/3))))
  Mux : Mux  Inputs=3
  vra_ref : Outport
  vrb_ref : Outport  Port=2
  vrc_ref : Outport  Port=3
  wires:
  vrd_ref/1 -> Mux/1
  vrq_ref/1 -> Mux/2
  Mux/1 -> Fcn1/1, Fcn/1, Fcn2/1
  Fcn/1 -> vra_ref/1
  Fcn1/1 -> vrb_ref/1
  Fcn2/1 -> vrc_ref/1
  téta_s/1 -> Mux/3

== system CommandeClassique/Subsystem/Subsystem ==
  Caer : Inport
  omega-mec : Inport  Port=2
  Gain : Gain  Gain=1/G
  Gain1 : Gain  Gain=1/G
  Cg : Outport
  omega-tur : Outport  Port=2
  wires:
  Caer/1 -> Gain/1
  Gain/1 -> Cg/1
  omega-mec/1 -> Gain1/1
  Gain1/1 -> omega-tur/1

== system CommandeClassique/Subsystem/Subsystem1 ==
  Cg : Inport
  Cem : Inport  Port=2
  Gain1 : Gain  Gain=1/J
  Gain4 : Gain  Gain=p
  Gain5 : Gain  Gain=F
  Integrator : Integrator  InitialCondition=32
  Sum : Sum  Inputs=|++-
  OMEGA : Outport
  w : Outport  Port=2
  wires:
  Integrator/1 -> OMEGA/1, Gain5/1, Gain4/1
  Gain1/1 -> Integrator/1
  Sum/1 -> Gain1/1
  Gain5/1 -> Sum/3
  Cg/1 -> Sum/1
  Cem/1 -> Sum/2
  Gain4/1 -> w/1

== system CommandeClassique/Subsystem/Subsystem3 ==
  e : Inport
  Gain : Gain  Gain=ki_mppt
  Gain1 : Gain  Gain=kp_mppt
  Gain2 : Gain  Gain=ki_mppt/kp_mppt
  Integrator : Integrator
  Saturation : Saturate  UpperLimit=1000  LowerLimit=-1000
  Sum : Sum  Inputs=|++
  Sum1 : Sum  Inputs=-|+
  Sum2 : Sum  Inputs=++|
  Imax : Outport
  wires:
  Sum1/1 -> Gain2/1
  Sum2/1 -> Gain/1
  Saturation/1 -> Sum1/2, Imax/1
  Gain1/1 -> Sum/2
  Integrator/1 -> Sum/1
  Gain/1 -> Integrator/1
  e/1 -> Sum2/2, Gain1/1
  Gain2/1 -> Sum2/1
  Sum/1 -> Saturation/1, Sum1/1

== system CommandeClassique/Subsystem/turbine ==
  omega_tur : Inport
  béta : Inport  Port=2
  V de vent : Inport  Port=3
  1/lamda-i : Fcn  Expr=(1/(u(2)+0.08*u(1)))-(0.035/(1+u(1)^3))
  Caer1 : Fcn  Expr=u(1)*((rou*s*u(3)^3)/2)*(1/u(2))
  Cp : Fcn  Expr=c1*(c2*u(1)-c3*u(2)-c4)*exp(-c5*u(1))+(c6/u(1))
  Mux : Mux  Inputs=2
  Mux1 : Mux  Inputs=2
  Mux2 : Mux  Inputs=2
  Mux3 : Mux  Inputs=3
  Scope1 : Scope
  Scope2 : Scope
  lamda : Fcn  Expr=u(1)*R/u(2)
  Caer : Outport
  wires:
  Mux/1 -> Cp/1
  Mux1/1 -> lamda/1
  omega_tur/1 -> Mux1/1, Mux3/2
  V de vent/1 -> Mux1/2, Mux3/3
  Mux2/1 -> 1/lamda-i/1
  lamda/1 -> Scope2/1, Mux2/2
  béta/1 -> Mux2/1, Mux/2
  1/lamda-i/1 -> Mux/1
  Mux3/1 -> Caer1/1
  Cp/1 -> Mux3/1, Scope1/1
  Caer1/1 -> Caer/1
